simulink model "Labormodell"  (R2013a)
settings: Solver=ode45  StartTime=0.0  StopTime=10.0  RelTol=1e-3
undefined symbols (not defined in the file): A_ss, b_ss, c_ss, q_max, q_min, v, w
settings Model: Creator=gonzalocastritius  LastModifiedBy=gonzalocastritius

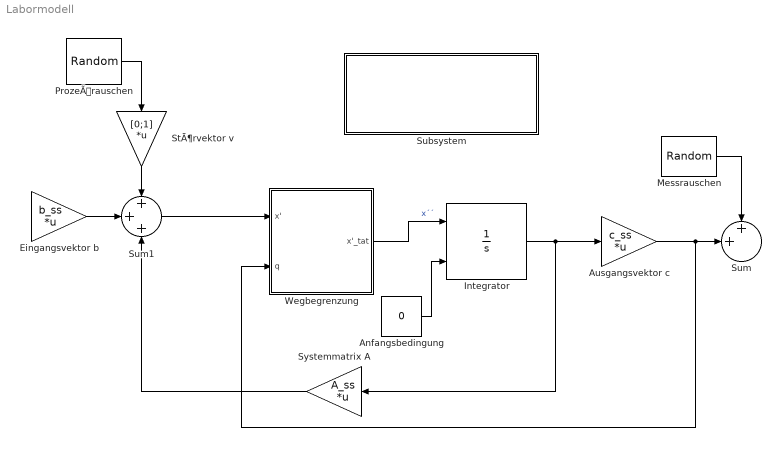
== system Labormodell ==
  Anfangsbedingung : Constant  Value=0
  Ausgangsvektor c : Gain  Gain=c_ss  Multiplication=Matrix(K*u)
  "Eingangsvektor b " : Gain  Gain=b_ss  Multiplication=Matrix(K*u)
  Integrator : Integrator  InitialConditionSource=external  UpperSaturationLimit=q_max  LowerSaturationLimit=q_min
  Messrauschen : RandomNumber  Variance=w  SampleTime=0.01
  ProzeÃrauschen : RandomNumber  Variance=v  SampleTime=0.01
  StÃ¶rvektor v : Gain  Gain=[0;1]  Multiplication=Matrix(K*u)
  Subsystem : Subsystem
      settings: OpenFcn=Parameter_Versuch
      mask Display: fprintf('Doppelclick um Parameter zu laden')
  Sum : Sum  Inputs=++|
  Sum1 : Sum  Inputs=+++
  Systemmatrix A : Gain  Gain=A_ss  Multiplication=Matrix(K*u)
  Wegbegrenzung : Subsystem
  wires:
  "Eingangsvektor b "/1 -> Sum1/2
  Anfangsbedingung/1 -> Integrator/2
  Ausgangsvektor c/1 -> Wegbegrenzung/2(q), Sum/2
  Integrator/1 -> Ausgangsvektor c/1, Systemmatrix A/1
  Wegbegrenzung/1(x'_tat) -> Integrator/1  "x´´"
  Sum1/1 -> Wegbegrenzung/1(x')
  Systemmatrix A/1 -> Sum1/3
  StÃ¶rvektor v/1 -> Sum1/1
  Messrauschen/1 -> Sum/1
  ProzeÃrauschen/1 -> StÃ¶rvektor v/1

== system Labormodell/Subsystem ==

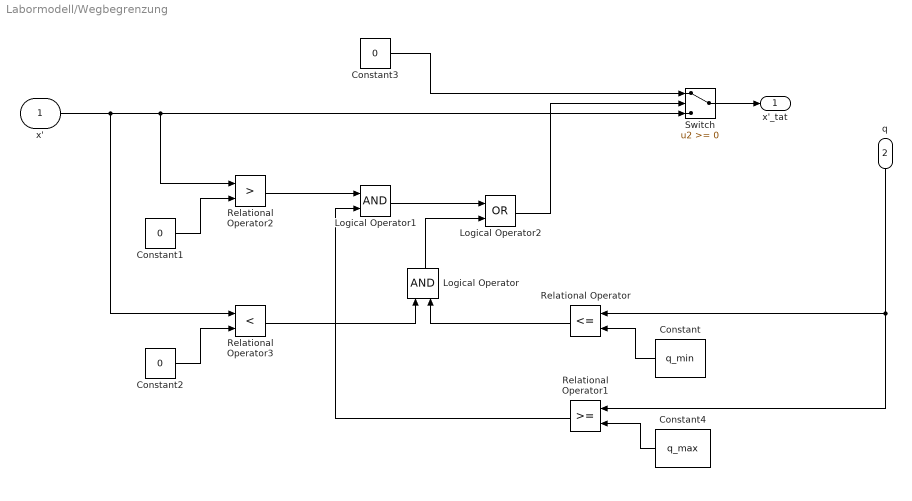
== system Labormodell/Wegbegrenzung ==
  x' : Inport
  q : Inport  Port=2
  Constant : Constant  Value=q_min
  Constant1 : Constant  Value=0
  Constant2 : Constant  Value=0
  Constant3 : Constant  Value=0
  Constant4 : Constant  Value=q_max
  Logical Operator : Logic  AllPortsSameDT=off  OutDataTypeStr=boolean
  Logical Operator1 : Logic  AllPortsSameDT=off  OutDataTypeStr=boolean
  Logical Operator2 : Logic  Operator=OR  AllPortsSameDT=off  OutDataTypeStr=boolean
  Relational Operator : RelationalOperator  Operator=<=  OutDataTypeStr=boolean
  Relational Operator1 : RelationalOperator  OutDataTypeStr=boolean
  Relational Operator2 : RelationalOperator  Operator=>  OutDataTypeStr=boolean
  Relational Operator3 : RelationalOperator  Operator=<  OutDataTypeStr=boolean
  Switch : Switch
  x'_tat : Outport
  wires:
  Relational Operator/1 -> Logical Operator/2
  x'/1 -> Relational Operator3/1, Relational Operator2/1, Switch/3
  Constant1/1 -> Relational Operator2/2
  Constant2/1 -> Relational Operator3/2
  Relational Operator2/1 -> Logical Operator1/1
  Relational Operator1/1 -> Logical Operator1/2
  Relational Operator3/1 -> Logical Operator/1
  Constant3/1 -> Switch/1
  Logical Operator/1 -> Logical Operator2/2
  Logical Operator1/1 -> Logical Operator2/1
  Logical Operator2/1 -> Switch/2
  Constant/1 -> Relational Operator/2
  Constant4/1 -> Relational Operator1/2
  Switch/1 -> x'_tat/1
  q/1 -> Relational Operator/1, Relational Operator1/1
